simulink model "FiltrosDigitais_01"  (R2018a)
settings: Solver=FixedStepDiscrete  StartTime=0.0  StopTime=0.1  FixedStep=50e-6  RelTol=1e-3
values from neighbouring files (symbols this model uses):
  fn = 50    [Basics_00_Param.m]
undefined symbols (not defined in the file or in its folder): Ts
libraries: PhD_Library x1, cstblocks x1, powerlib_meascontrol x1
settings Model: Creator=daniemot  LastModifiedBy=daniemot

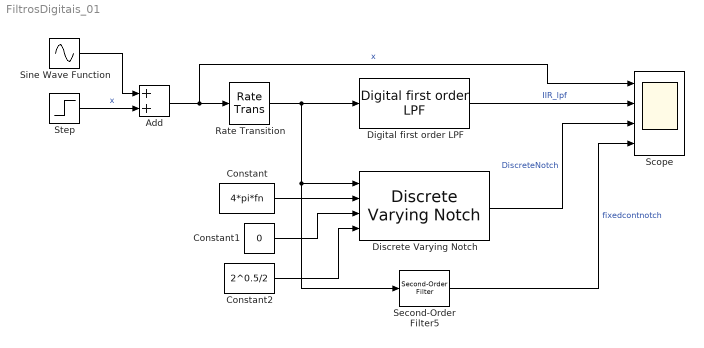
== system FiltrosDigitais_01 ==
  Add : Sum
  Constant : Constant  Value=4*pi*fn
  Constant1 : Constant  Value=0
  Constant2 : Constant  Value=2^0.5/2
  Digital first order LPF : PhD_Library/Offshore_Oil_and_Wind/Digital first order LPF  Ts=Ts  fcutout=fn/2^0.5
  Discrete Varying Notch : cstblocks/Linear Parameter Varying/Discrete Varying Notch  w0=0  Ts=Ts
      settings: SourceProductName=Control System Toolbox  SourceProductBaseCode=CT
  Rate Transition : RateTransition  OutPortSampleTime=Ts
  Scope : Scope  NumInputPorts=4
  Second-Order Filter5 : powerlib_meascontrol/Filters/Second-Order Filter  FilterType=Bandstop (Notch)  Fo=2*fn  Zeta=2^0.5/2  Ts=Ts  Initialize=off  Vac_Init="[0,  0,  60]"  Vdc_Init=0  PlotResponse=off  FreqRange=[0, 1000, 0.1]
      settings: SourceProductName=Simscape Power Systems  SourceProductBaseCode=PS
  Sine Wave Function : Sin  Frequency=4*pi*fn  SampleTime=0
  Step : Step  Time=100000  After=2  SampleTime=0
  wires:
  Add/1 -> Scope/1, Rate Transition/1  "x"
  Step/1 -> Add/2  "x"
  Sine Wave Function/1 -> Add/1
  Digital first order LPF/1 -> Scope/2  "IIR_lpf"
  Rate Transition/1 -> Second-Order Filter5/1, Discrete Varying Notch/1, Digital first order LPF/1
  Constant/1 -> Discrete Varying Notch/2
  Constant1/1 -> Discrete Varying Notch/3
  Constant2/1 -> Discrete Varying Notch/4
  Discrete Varying Notch/1 -> Scope/3  "DiscreteNotch"
  Second-Order Filter5/1 -> Scope/4  "fixedcontnotch"
